simulink model "Detumbling1"  (R2024a)
settings: Solver=ode4  StartTime=0.0  StopTime=1000  FixedStep=0.001  RelTol=1e-3
settings Model: Creator=jsa102  LastModifiedBy=maria
settings RTWCC: GPUComputeCapability=3.5

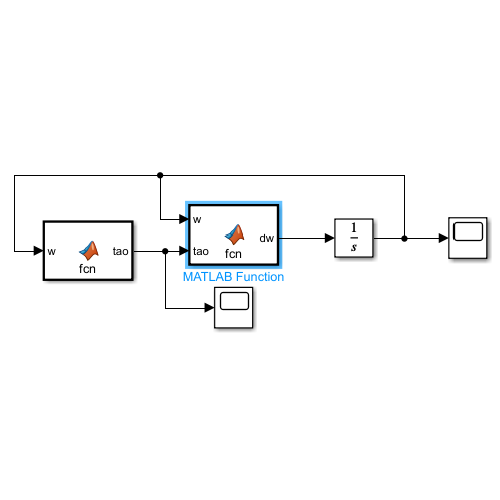
[thumbnail: Simulink's stored preview of the top-level diagram]
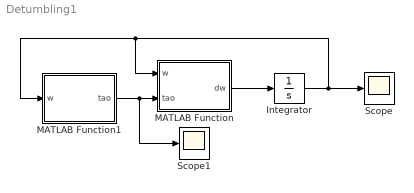
== system Detumbling1 ==
  Integrator : Integrator  InitialCondition=[0; 0; 2*pi*1]
  MATLAB Function : MATLAB Function  TreatAsAtomicUnit=on
  MATLAB Function1 : MATLAB Function  TreatAsAtomicUnit=on
  Scope : Scope
  Scope1 : Scope
  wires:
  MATLAB Function/1(dw) -> Integrator/1
  Integrator/1 -> Scope/1, MATLAB Function1/1(w), MATLAB Function/1(w)
  MATLAB Function1/1(tao) -> Scope1/1, MATLAB Function/2(tao)

== matlab function Detumbling1/MATLAB Function ==
  data: w input; tao input; dw output
function dw  = fcn(w,tao)

m = 2.66;
%a = 0.1;
%b = 0.1;
%c = 0.2;

Jxx = 1/12*m*(0.1^2+0.2^2);
Jyy = 1/12*m*(0.2^2+0.1^2);
Jzz = 1/12*m*(0.1^2+0.1^2);
%parallel theorem 

J = [Jxx 0 0;
     0 Jyy 0;
     0 0 Jzz];

%J = ((1/6)*m*a^2)*eye(3);

dw = inv(J)*(tao - cross(w,J*w));

%Nex step: have total torque and have the magnetorques model (each one)

== matlab function Detumbling1/MATLAB Function1 ==
  data: w input; tao output
function tao = fcn(w)

kd = -1;

% max_magtorq = 250e-6; %Maximum value
% cm = [0 0 0]; %Center of mass
% loc_magtorq_1 = [0 0.04 0.8]; 
% loc_magtorq_2 = [0.4 0 0.8]; 
% 
% tao_vec_x = max_magtorq*tanh(kd*w)*(loc_magtorq_1-cm);
% tao_vec_y = max_magtorq*tanh(kd*w)*(loc_magtorq_2-cm);
% tao_vec = tao_vec_x + tao_vec_y;
% %n_mt_axis = 1; %Number of magnetorquers in axis x and y 
% %tao_vec = n_mt_axis*max_magtorq*(tanh(kd*w)*abs(loc_magtorq_1-cm));
% tao = -norm(tao_vec);


tao = 450e-06*tanh(kd*w); %450 will be the max produced by each magnetorquer


%torque = m X B
